simulink model "HFI_Test"  (R2023a)
settings: Solver=FixedStepAuto  StartTime=0.0  StopTime=1  FixedStep=Ts_simulink  RelTol=1e-3
model workspace (MATLAB code in the model file):
  | cmdLim = Simulink.Parameter;
  | cmdLim.Value = 15;
  | cmdLim.Description = 'Limit for controlling the maximum surface command angle.';
  | cmdLim.Min = 0;
  | cmdLim.Max = 90;
  | cmdLim.DocUnits = 'deg';
  | 
  | dispGain = Simulink.Parameter;
  | dispGain.Value = 0.75;
  | dispGain.Description = 'Gain applied to the displacement error.';
  | dispGain.Min = 0;
  | dispGain.Max = [];
  | dispGain.DocUnits = 'deg/sec/deg';
  | 
  | dispLim = Simulink.Parameter;
  | dispLim.Value = 30;
  | dispLim.Description = 'Limit for controlling the maximum commanded angle.';
  | dispLim.Min = 0;
  | dispLim.Max = 180;
  | dispLim.DocUnits = 'deg';
  | 
  | intGain = Simulink.Parameter;
  | intGain.Value = 0.5;
  | intGain.Description = 'Gain applied to the integral error.';
  | intGain.Min = 0;
  | intGain.Max = [];
  | intGain.DocUnits = 'deg/sec/deg/sec';
  | 
  | intLim = Simulink.Parameter;
  | intLim.Value = 5;
  | intLim.Description = 'Limit for controlling the maximum commanded angle.';
  | intLim.Min = 0;
  | intLim.Max = 90;
  | intLim.DocUnits = 'deg';
  | 
  | rateGain = Simulink.Parameter;
  | rateGain.Value = 2;
  | rateGain.Description = 'Gain applied to the rate error.';
  | rateGain.Min = 0;
  | rateGain.Max = [];
  | rateGain.DocUnits = 'deg/deg/sec';
  | 
  | rateLim = Simulink.Parameter;
  | rateLim.Value = 6;
  | rateLim.Description = 'Limit for controlling the maximum commanded angle.';
  | rateLim.Min = 0;
  | rateLim.Max = 180;
  | rateLim.DocUnits = 'deg/sec';
  | 
  | hdgGain = Simulink.Parameter;
  | hdgGain.Value = 0.015;
undefined symbols (not defined in the file): inverter, pmsm, Ts_motor, Ts_simulink
libraries: mcbcontrolslib x3, autolibpmsminterior x1, mcbplantlib x1
settings Model: RequirementInfo={} %GIDa_fe9045fd_0412_4b6e_8206_617cc20e6fde  Creator=洲  LastModifiedBy=洲
settings SolverCC: AlgebraicLoopSolver=TrustRegion  AutoInsertRateTranBlk=on
settings DataIOCC: SaveOutput=off  DSMLogging=off  SaveTime=off
settings OptimizationCC: DefaultParameterBehavior=Inlined  UseDivisionForNetSlopeComputation=on  GainParamInheritBuiltInType=on  UseFloatMulNetSlope=on  UseSpecifiedMinMax=on  InlineInvariantSignals=on  EnhancedBackFolding=on  PassReuseOutputArgsAs=Individual arguments  ZeroExternalMemoryAtStartup=off  ZeroInternalMemoryAtStartup=off  NoFixptDivByZeroProtection=on  EfficientFloat2IntCast=on  LifeSpan=1  OptimizeBlockOrder=speed  DifferentSizesBufferReuse=on  OptimizationCustomize=off  EfficientTunableParamExpr=on
settings DebuggingCC: AllowSymbolicDim=off  SFUnexpectedBacktrackingDiag=warning  SFNoUnconditionalDefaultTransitionDiag=warning  SFExecutionAtInitializationDiag=none  ArithmeticOperatorsInVariantConditions=warning
settings HardwareCC: ProdLongLongMode=on
settings SFSimCC: MATLABDynamicMemAlloc=off
settings RTWCC: Description=Embedded Coder  SystemTargetFile=ert.tlc  TemplateMakefile=ert_default_tmf  BuildConfiguration=Faster Runs  DataTypeReplacement=CDataTypesFixedWidth
settings CodeAppCC: ForceParamTrailComments=on  IgnoreCustomStorageClasses=off  OperatorAnnotations=on  SimulinkDataObjDesc=on  SFDataObjDesc=on  CustomSymbolStrGlobalVar=rt$N$M  CustomSymbolStrType=$N$M  CustomSymbolStrFcn=$N$M$F  CustomSymbolStrMacro=$N$M  InsertBlockDesc=on  EnableCustomComments=on  ReqsInCode=on
settings ERTTargetCC: TargetLangStandard=C99 (ISO)  UtilityFuncGeneration=Shared location  MultiwordLength=2048  GenerateSampleERTMain=on  IncludeMdlTerminateFcn=off  CombineSignalStateStructs=on  SuppressErrorStatus=on  SupportAbsoluteTime=off  SupportNonFinite=off  SupportComplex=off  InlinedParameterPlacement=NonHierarchical  ERTCustomFileTemplate=example_file_process.tlc  ERTFilePackagingFormat=CompactWithDataFile
settings ConfigComp: CovScope=ReferencedModels  CovSaveName=covdata_rollAP  CovMetricSettings=dcmtrwe  CovHTMLOptions=-sRT=1 -aTS=1 -bRG=1 -bTC=1 -hTR=1 -nFC=0 -scm=1 -bcm=1 -xEv=0  CovSaveCumulativeToWorkspaceVar=on  CovSaveSingleToWorkspaceVar=on  CovCumulativeVarName=covCumulativeData_rollAP  CovReportOnPause=off  CovExternalEMLEnable=off  CovSFcnEnable=off

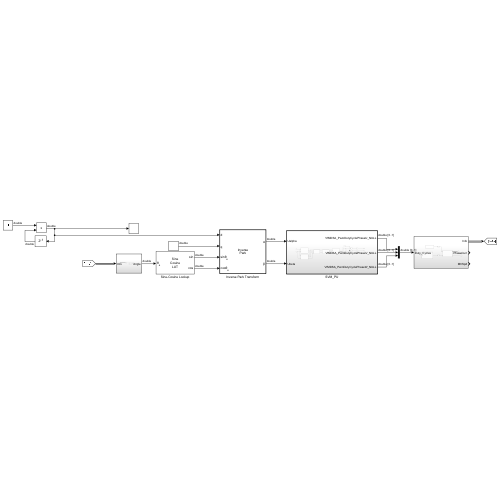
[thumbnail: Simulink's stored preview of the top-level diagram]
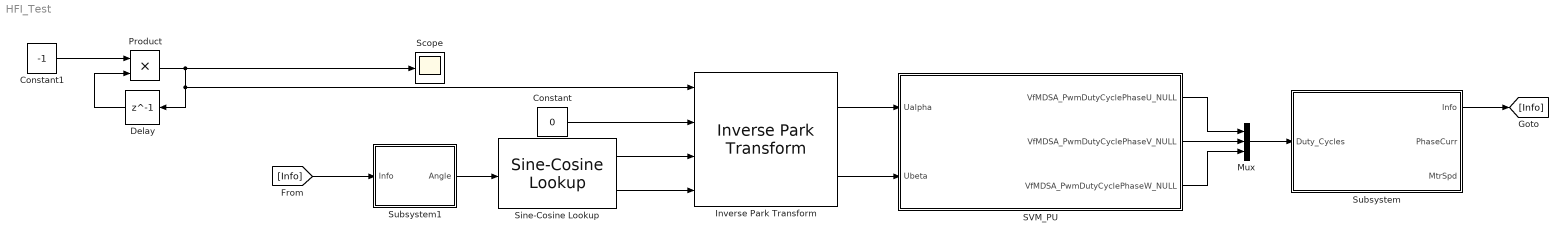
== system HFI_Test ==
  Constant : Constant  Value=0
  Constant1 : Constant  Value=-1  SampleTime=1e-4
  Delay : Delay  DelayLength=1  InitialCondition=3
  Inverse Park Transform : mcbcontrolslib/Inverse Park Transform  AxisAlignment=D-axis
      settings: LibrarySourceBlock=mcblib/Controls/Math Transforms/Inverse Park Transform
  Mux : Mux  Inputs=3
  Product : Product
  SVM_PU : Subsystem  TreatAsAtomicUnit=on  RTWFcnName=SVPWM_Calc
      settings: RTWSystemCode=Nonreusable function  RTWFcnNameOpts=User specified
  Scope : Scope
  Sine-Cosine Lookup : mcbcontrolslib/Sine-Cosine Lookup  AngleInput=Radians  N_points=4095
      settings: LibrarySourceBlock=mcblib/Controls/Math Transforms/Sine-Cosine Lookup
  Subsystem : Subsystem
  Subsystem1 : Subsystem
  wires:
  Mux/1 -> Subsystem/1(Duty_Cycles)
  SVM_PU/2(VfMDSA_PwmDutyCyclePhaseV_NULL) -> Mux/2
  SVM_PU/1(VfMDSA_PwmDutyCyclePhaseU_NULL) -> Mux/1
  SVM_PU/3(VfMDSA_PwmDutyCyclePhaseW_NULL) -> Mux/3
  Inverse Park Transform/1 -> SVM_PU/1(Ualpha)
  Inverse Park Transform/2 -> SVM_PU/2(Ubeta)
  Subsystem/1(Info) -> [Info]
  Sine-Cosine Lookup/2 -> Inverse Park Transform/4
  Sine-Cosine Lookup/1 -> Inverse Park Transform/3
  [Info] -> Subsystem1/1(Info)
  Subsystem1/1(Angle) -> Sine-Cosine Lookup/1
  Constant/1 -> Inverse Park Transform/2
  Product/1 -> Inverse Park Transform/1, Delay/1, Scope/1
  Delay/1 -> Product/2
  Constant1/1 -> Product/1

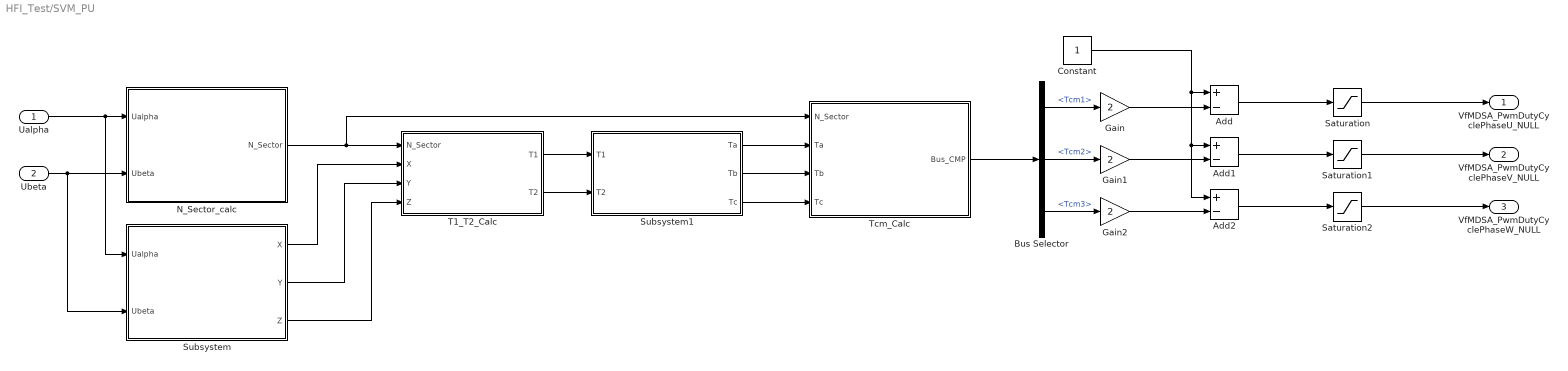
== system HFI_Test/SVM_PU ==
  Ualpha : Inport
  Ubeta : Inport  Port=2
  Add : Sum  Inputs=+-
  Add1 : Sum  Inputs=+-
  Add2 : Sum  Inputs=+-
  Bus Selector : BusSelector  OutputSignals=Tcm1,Tcm2,Tcm3
  Constant : Constant  OutDataTypeStr=single
  Gain : Gain  Gain=2
  Gain1 : Gain  Gain=2
  Gain2 : Gain  Gain=2
  N_Sector_calc : Subsystem
  Saturation : Saturate  UpperLimit=1  LowerLimit=0
  Saturation1 : Saturate  UpperLimit=1  LowerLimit=0
  Saturation2 : Saturate  UpperLimit=1  LowerLimit=0
  Subsystem : Subsystem
  Subsystem1 : Subsystem
  T1_T2_Calc : Subsystem
  Tcm_Calc : Subsystem
  VfMDSA_PwmDutyCyclePhaseU_NULL : Outport  OutMin=0  OutMax=1
  VfMDSA_PwmDutyCyclePhaseV_NULL : Outport  Port=2  OutMin=0  OutMax=1
  VfMDSA_PwmDutyCyclePhaseW_NULL : Outport  Port=3  OutMin=0  OutMax=1
  wires:
  Ualpha/1 -> Subsystem/1(Ualpha), N_Sector_calc/1(Ualpha)
  Ubeta/1 -> Subsystem/2(Ubeta), N_Sector_calc/2(Ubeta)
  N_Sector_calc/1(N_Sector) -> Tcm_Calc/1(N_Sector), T1_T2_Calc/1(N_Sector)
  Subsystem/1(X) -> T1_T2_Calc/2(X)
  Subsystem/2(Y) -> T1_T2_Calc/3(Y)
  Subsystem/3(Z) -> T1_T2_Calc/4(Z)
  Subsystem1/1(Ta) -> Tcm_Calc/2(Ta)
  Subsystem1/2(Tb) -> Tcm_Calc/3(Tb)
  Subsystem1/3(Tc) -> Tcm_Calc/4(Tc)
  Tcm_Calc/1(Bus_CMP) -> Bus Selector/1
  T1_T2_Calc/1(T1) -> Subsystem1/1(T1)
  T1_T2_Calc/2(T2) -> Subsystem1/2(T2)
  Bus Selector/1 -> Gain/1  "<Tcm1>"
  Bus Selector/2 -> Gain1/1  "<Tcm2>"
  Bus Selector/3 -> Gain2/1  "<Tcm3>"
  Constant/1 -> Add2/1, Add1/1, Add/1
  Gain/1 -> Add/2
  Gain1/1 -> Add1/2
  Gain2/1 -> Add2/2
  Add/1 -> Saturation/1
  Add1/1 -> Saturation1/1
  Add2/1 -> Saturation2/1
  Saturation/1 -> VfMDSA_PwmDutyCyclePhaseU_NULL/1
  Saturation1/1 -> VfMDSA_PwmDutyCyclePhaseV_NULL/1
  Saturation2/1 -> VfMDSA_PwmDutyCyclePhaseW_NULL/1

== system HFI_Test/Subsystem ==
  Duty_Cycles : Inport
  Interior PMSM : autolibpmsminterior/Interior PMSM  port_config=Torque  sim_type=Discrete  Ts=Ts_motor  P=4  Rs=0.02  Ldq=[1.7e-3 3.2e-3]  KConstText=Permanent flux linkage constant (lambda_pm):  lambda_pm=0.2205  Ke=159.9771  mechanical=[0.002700,4.924e-4,0]  idq0=[0 0]  theta_init=0  omega_init=0  KConst=0.2205  lambda_pm_calc=0.2205  Kt=0.07  RefBlkName='autolibpmsminterior/Interior PMSM'  aMode=5
      settings: LibrarySourceBlock=mcblib/Electrical Systems/Motors/Interior PMSM
  Inverter : Subsystem
  Load_Profile (Torque) : Subsystem
  Rate Transition : RateTransition  Deterministic=off  OutPortSampleTime=Ts_motor
  Rate Transition1 : RateTransition  Deterministic=off  OutPortSampleTime=Ts_motor
  Info : Outport
  PhaseCurr : Outport  Port=2
  MtrSpd : Outport  Port=3
  wires:
  Inverter/1(Vabc) -> Rate Transition/1  "Vabc"
  Rate Transition1/1 -> Interior PMSM/1
  Interior PMSM/3 -> MtrSpd/1
  Duty_Cycles/1 -> Inverter/1(Duty_abc)
  Rate Transition/1 -> Interior PMSM/2
  Interior PMSM/2 -> PhaseCurr/1  "Iabc"
  Load_Profile (Torque)/1(Load_Trq) -> Rate Transition1/1
  Interior PMSM/1 -> Info/1

== system HFI_Test/Subsystem1 ==
  Info : Inport
  Bus Selector : BusSelector  OutputSignals=MtrPos
  Constant : Constant  Value=2*pi
  Gain : Gain  Gain=4
  Mod : Math  Operator=mod
  Angle : Outport
  wires:
  Gain/1 -> Mod/1
  Mod/1 -> Angle/1
  Bus Selector/1 -> Gain/1  "<MtrPos>"
  Constant/1 -> Mod/2
  Info/1 -> Bus Selector/1

== system HFI_Test/SVM_PU/N_Sector_calc ==
  Ualpha : Inport
  Ubeta : Inport  Port=2
  N_calc : Subsystem
  Uref_Calc : Subsystem
  N_Sector : Outport
  wires:
  Uref_Calc/2(Uref2) -> N_calc/2(Uref2)
  Ualpha/1 -> Uref_Calc/1(Ualpha)
  Ubeta/1 -> Uref_Calc/2(Ubeta)
  Uref_Calc/3(Uref3) -> N_calc/3(Uref3)
  N_calc/1(N_Sector) -> N_Sector/1
  Uref_Calc/1(Uref1) -> N_calc/1(Uref1)

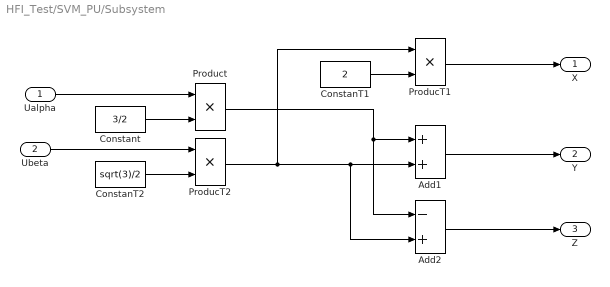
== system HFI_Test/SVM_PU/Subsystem ==
  Ualpha : Inport
  Ubeta : Inport  Port=2
  Add1 : Sum
  Add2 : Sum  Inputs=-+
  ConstanT1 : Constant  Value=2  OutDataTypeStr=single
  ConstanT2 : Constant  Value=sqrt(3)/2  OutDataTypeStr=single
  Constant : Constant  Value=3/2  OutDataTypeStr=single
  ProducT1 : Product
  ProducT2 : Product
  Product : Product
  X : Outport
  Y : Outport  Port=2
  Z : Outport  Port=3
  wires:
  Ualpha/1 -> Product/1
  Constant/1 -> Product/2
  ProducT1/1 -> X/1
  ConstanT1/1 -> ProducT1/2
  Ubeta/1 -> ProducT2/1
  Add1/1 -> Y/1
  Product/1 -> Add2/1, Add1/1
  ProducT2/1 -> ProducT1/1, Add2/2, Add1/2
  ConstanT2/1 -> ProducT2/2
  Add2/1 -> Z/1

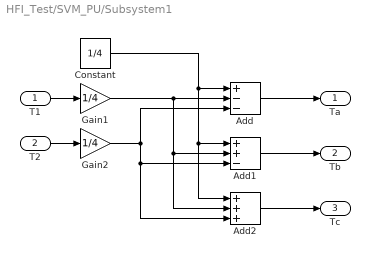
== system HFI_Test/SVM_PU/Subsystem1 ==
  T1 : Inport
  T2 : Inport  Port=2
  Add : Sum  Inputs=+--
  Add1 : Sum  Inputs=++-
  Add2 : Sum  Inputs=+++
  Constant : Constant  Value=1/4  OutDataTypeStr=single
  Gain1 : Gain  Gain=1/4
  Gain2 : Gain  Gain=1/4
  Ta : Outport
  Tb : Outport  Port=2
  Tc : Outport  Port=3
  wires:
  T1/1 -> Gain1/1
  T2/1 -> Gain2/1
  Constant/1 -> Add2/1, Add1/1, Add/1
  Add/1 -> Ta/1
  Gain1/1 -> Add2/2, Add1/2, Add/2
  Gain2/1 -> Add1/3, Add2/3, Add/3
  Add1/1 -> Tb/1
  Add2/1 -> Tc/1

== system HFI_Test/SVM_PU/T1_T2_Calc ==
  N_Sector : Inport
  X : Inport  Port=2
  Y : Inport  Port=3
  Z : Inport  Port=4
  Subsystem1 : Subsystem
  Subsystem2 : Subsystem
  T4_T6 : Subsystem  Commented=on
  T1 : Outport
  T2 : Outport  Port=2
  wires:
  X/1 -> Subsystem1/2(X)
  Z/1 -> Subsystem1/4(Z)
  N_Sector/1 -> Subsystem1/1(N_Sector)
  Y/1 -> Subsystem1/3(Y)
  Subsystem1/1(Bus_T4T6) -> Subsystem2/1(Bus_T4T6)
  Subsystem2/1(T1) -> T1/1
  Subsystem2/2(T2) -> T2/1

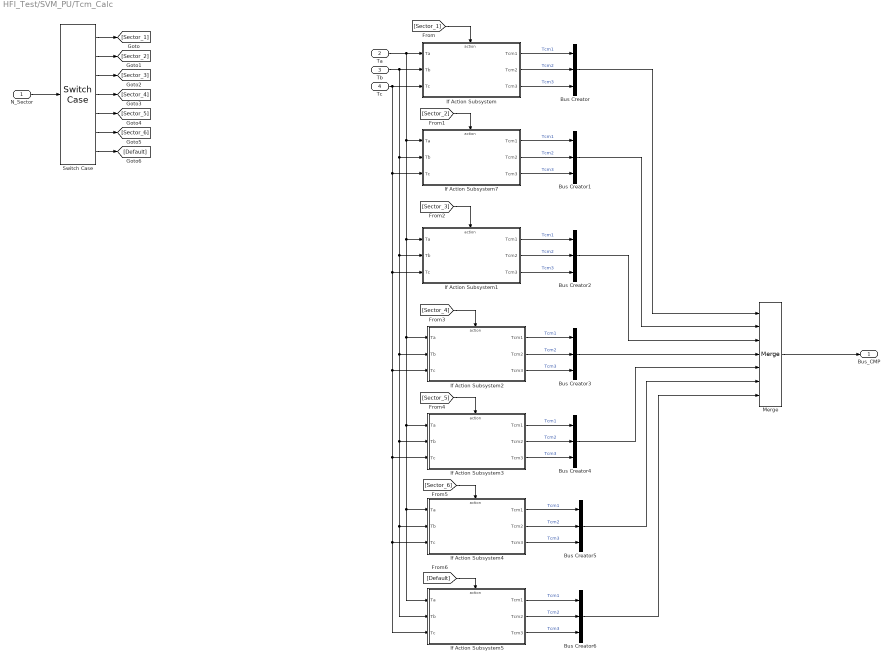
== system HFI_Test/SVM_PU/Tcm_Calc ==
  N_Sector : Inport
  Ta : Inport  Port=2
  Tb : Inport  Port=3
  Tc : Inport  Port=4
  Bus Creator{,1..6} (7 alike) : BusCreator  Inputs=3
  If Action Subsystem : Subsystem  TreatAsAtomicUnit=on
  If Action Subsystem1 : Subsystem  TreatAsAtomicUnit=on
  If Action Subsystem2 : Subsystem  TreatAsAtomicUnit=on
  If Action Subsystem3 : Subsystem  TreatAsAtomicUnit=on
  If Action Subsystem4 : Subsystem  TreatAsAtomicUnit=on
  If Action Subsystem5 : Subsystem  TreatAsAtomicUnit=on
  If Action Subsystem7 : Subsystem  TreatAsAtomicUnit=on
  Merge : Merge  Inputs=7
  Switch Case : SwitchCase  CaseConditions={1,2,3,4,5,6}
  Bus_CMP : Outport
  wires:
  Switch Case/1 -> [Sector_1]
  Switch Case/2 -> [Sector_2]
  Switch Case/4 -> [Sector_4]
  Switch Case/6 -> [Sector_6]
  Switch Case/3 -> [Sector_3]
  N_Sector/1 -> Switch Case/1
  Switch Case/7 -> [Default]
  Switch Case/5 -> [Sector_5]
  [Sector_1] -> If Action Subsystem/Action
  [Sector_2] -> If Action Subsystem7/Action
  [Sector_4] -> If Action Subsystem2/Action
  [Sector_3] -> If Action Subsystem1/Action
  [Sector_6] -> If Action Subsystem4/Action
  [Sector_5] -> If Action Subsystem3/Action
  [Default] -> If Action Subsystem5/Action
  Tb/1 -> If Action Subsystem5/2(Tb), If Action Subsystem4/2(Tb), If Action Subsystem3/2(Tb), If Action Subsystem2/2(Tb), If Action Subsystem1/2(Tb), If Action Subsystem7/2(Tb), If Action Subsystem/2(Tb)
  Tc/1 -> If Action Subsystem/3(Tc), If Action Subsystem5/3(Tc), If Action Subsystem4/3(Tc), If Action Subsystem3/3(Tc), If Action Subsystem2/3(Tc), If Action Subsystem1/3(Tc), If Action Subsystem7/3(Tc)
  Ta/1 -> If Action Subsystem5/1(Ta), If Action Subsystem4/1(Ta), If Action Subsystem3/1(Ta), If Action Subsystem2/1(Ta), If Action Subsystem1/1(Ta), If Action Subsystem7/1(Ta), If Action Subsystem/1(Ta)
  Merge/1 -> Bus_CMP/1
  If Action Subsystem/1(Tcm1) -> Bus Creator/1  "Tcm1"
  If Action Subsystem/2(Tcm2) -> Bus Creator/2  "Tcm2"
  If Action Subsystem/3(Tcm3) -> Bus Creator/3  "Tcm3"
  If Action Subsystem7/1(Tcm1) -> Bus Creator1/1  "Tcm1"
  If Action Subsystem7/3(Tcm3) -> Bus Creator1/3  "Tcm3"
  If Action Subsystem7/2(Tcm2) -> Bus Creator1/2  "Tcm2"
  If Action Subsystem1/1(Tcm1) -> Bus Creator2/1  "Tcm1"
  If Action Subsystem1/3(Tcm3) -> Bus Creator2/3  "Tcm3"
  If Action Subsystem1/2(Tcm2) -> Bus Creator2/2  "Tcm2"
  If Action Subsystem2/1(Tcm1) -> Bus Creator3/1  "Tcm1"
  If Action Subsystem2/3(Tcm3) -> Bus Creator3/3  "Tcm3"
  If Action Subsystem2/2(Tcm2) -> Bus Creator3/2  "Tcm2"
  If Action Subsystem3/1(Tcm1) -> Bus Creator4/1  "Tcm1"
  If Action Subsystem3/3(Tcm3) -> Bus Creator4/3  "Tcm3"
  If Action Subsystem3/2(Tcm2) -> Bus Creator4/2  "Tcm2"
  If Action Subsystem4/1(Tcm1) -> Bus Creator5/1  "Tcm1"
  If Action Subsystem4/3(Tcm3) -> Bus Creator5/3  "Tcm3"
  If Action Subsystem4/2(Tcm2) -> Bus Creator5/2  "Tcm2"
  If Action Subsystem5/1(Tcm1) -> Bus Creator6/1  "Tcm1"
  If Action Subsystem5/3(Tcm3) -> Bus Creator6/3  "Tcm3"
  If Action Subsystem5/2(Tcm2) -> Bus Creator6/2  "Tcm2"
  Bus Creator/1 -> Merge/1
  Bus Creator1/1 -> Merge/2
  Bus Creator2/1 -> Merge/3
  Bus Creator3/1 -> Merge/4
  Bus Creator4/1 -> Merge/5
  Bus Creator5/1 -> Merge/6
  Bus Creator6/1 -> Merge/7

== system HFI_Test/Subsystem/Inverter ==
  Duty_abc : Inport
  Average-Value Inverter : mcbplantlib/Average-Value Inverter
  Constant2 : Constant  Value=inverter.V_dc  OutDataTypeStr=single  SampleTime=-1
  Data Type Conversion1 : DataTypeConversion  OutDataTypeStr=single  RndMeth=Simplest  SaturateOnIntegerOverflow=off
  Rate Transition3 : RateTransition  Deterministic=off  OutPortSampleTime=Ts_inverter
  Vabc : Outport  VectorParamsAs1DForOutWhenUnconnected=off
  wires:
  Constant2/1 -> Average-Value Inverter/2
  Data Type Conversion1/1 -> Rate Transition3/1
  Duty_abc/1 -> Data Type Conversion1/1
  Average-Value Inverter/1 -> Vabc/1
  Rate Transition3/1 -> Average-Value Inverter/1

== system HFI_Test/Subsystem/Load_Profile (Torque) ==
  Constant : Constant  Value=0
  Data Type Conversion : DataTypeConversion  OutDataTypeStr=single  SaturateOnIntegerOverflow=off  RndMeth=Floor
  IIR Filter : mcbcontrolslib/IIR Filter  VariantControl=Low Pass Filter  VariantSelect=Low-pass  Filter_constant=0.0001  advancedSettings=off  Ts=50e-6  cutOff_freq=0.31834
  T_load : Step  Commented=on  Time=4  Before=0.05*pmsm.T_rated  After=0.5*pmsm.T_rated  SampleTime=Ts_simulink
  Load_Trq : Outport  VectorParamsAs1DForOutWhenUnconnected=off
  wires:
  Data Type Conversion/1 -> IIR Filter/1
  IIR Filter/1 -> Load_Trq/1
  Constant/1 -> Data Type Conversion/1

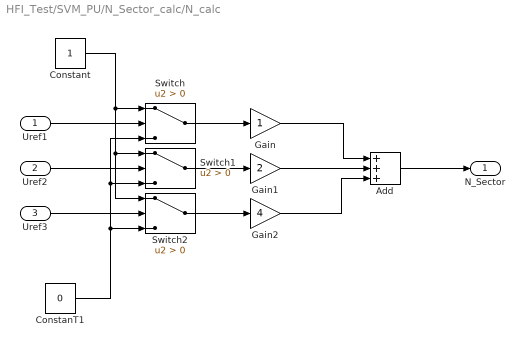
== system HFI_Test/SVM_PU/N_Sector_calc/N_calc ==
  Uref1 : Inport
  Uref2 : Inport  Port=2
  Uref3 : Inport  Port=3
  Add : Sum  Inputs=+++
  ConstanT1 : Constant  Value=0  OutDataTypeStr=single
  Constant : Constant  OutDataTypeStr=single
  Gain : Gain
  Gain1 : Gain  Gain=2
  Gain2 : Gain  Gain=4
  Switch : Switch  Criteria=u2 > Threshold  SaturateOnIntegerOverflow=off  InputSameDT=off
  Switch1 : Switch  Criteria=u2 > Threshold  SaturateOnIntegerOverflow=off  InputSameDT=off
  Switch2 : Switch  Criteria=u2 > Threshold  SaturateOnIntegerOverflow=off  InputSameDT=off
  N_Sector : Outport
  wires:
  Uref1/1 -> Switch/2
  Uref2/1 -> Switch1/2
  Uref3/1 -> Switch2/2
  ConstanT1/1 -> Switch2/3, Switch/3, Switch1/3
  Constant/1 -> Switch2/1, Switch1/1, Switch/1
  Switch1/1 -> Gain1/1
  Switch/1 -> Gain/1
  Switch2/1 -> Gain2/1
  Add/1 -> N_Sector/1
  Gain/1 -> Add/1
  Gain1/1 -> Add/2
  Gain2/1 -> Add/3

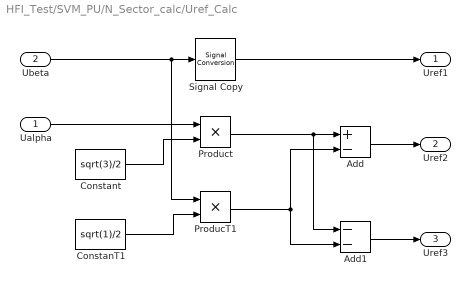
== system HFI_Test/SVM_PU/N_Sector_calc/Uref_Calc ==
  Ualpha : Inport
  Ubeta : Inport  Port=2
  Add : Sum  Inputs=+-
  Add1 : Sum  Inputs=--
  ConstanT1 : Constant  Value=sqrt(1)/2  OutDataTypeStr=single
  Constant : Constant  Value=sqrt(3)/2  OutDataTypeStr=single
  ProducT1 : Product
  Product : Product
  Signal Copy : SignalConversion  OverrideOpt=off
  Uref1 : Outport
  Uref2 : Outport  Port=2
  Uref3 : Outport  Port=3
  wires:
  Ubeta/1 -> ProducT1/1, Signal Copy/1
  Signal Copy/1 -> Uref1/1
  Ualpha/1 -> Product/1
  Constant/1 -> Product/2
  ConstanT1/1 -> ProducT1/2
  Product/1 -> Add1/1, Add/1
  ProducT1/1 -> Add1/2, Add/2
  Add/1 -> Uref2/1
  Add1/1 -> Uref3/1

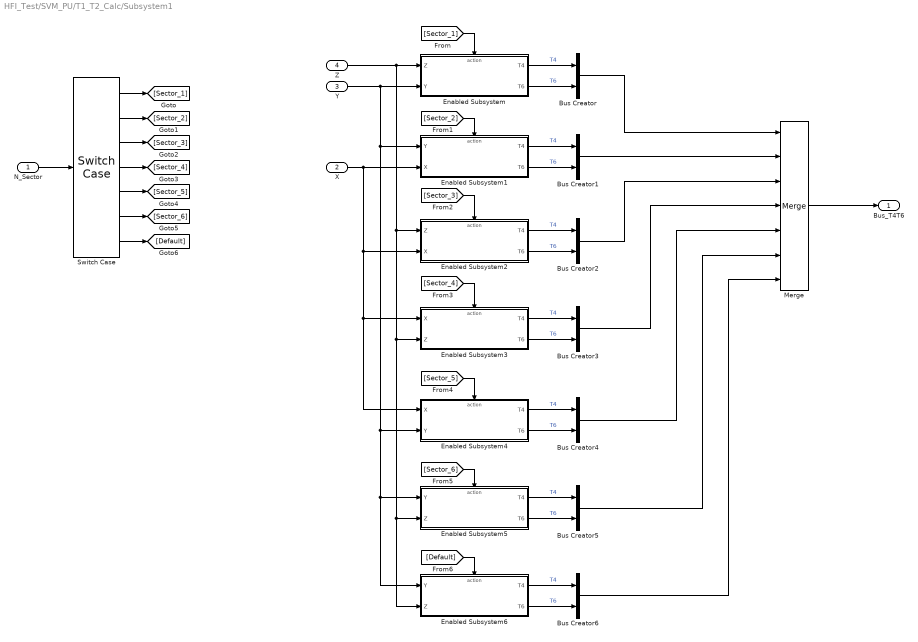
== system HFI_Test/SVM_PU/T1_T2_Calc/Subsystem1 ==
  N_Sector : Inport
  X : Inport  Port=2
  Y : Inport  Port=3
  Z : Inport  Port=4
  Bus Creator{,1..6} (7 alike) : BusCreator  Inputs=2
  Enabled Subsystem : Subsystem  TreatAsAtomicUnit=on
  Enabled Subsystem1 : Subsystem  TreatAsAtomicUnit=on
  Enabled Subsystem2 : Subsystem  TreatAsAtomicUnit=on
  Enabled Subsystem3 : Subsystem  TreatAsAtomicUnit=on
  Enabled Subsystem4 : Subsystem  TreatAsAtomicUnit=on
  Enabled Subsystem5 : Subsystem  TreatAsAtomicUnit=on
  Enabled Subsystem6 : Subsystem  TreatAsAtomicUnit=on
  Merge : Merge  Inputs=7
  Switch Case : SwitchCase  CaseConditions={1,2,3,4,5,6}
  Bus_T4T6 : Outport
  wires:
  N_Sector/1 -> Switch Case/1
  Switch Case/1 -> [Sector_1]
  Switch Case/2 -> [Sector_2]
  Switch Case/3 -> [Sector_3]
  Switch Case/4 -> [Sector_4]
  Switch Case/5 -> [Sector_5]
  Switch Case/6 -> [Sector_6]
  Switch Case/7 -> [Default]
  [Sector_1] -> Enabled Subsystem/Action
  Y/1 -> Enabled Subsystem6/1(Y), Enabled Subsystem5/1(Y), Enabled Subsystem4/2(Y), Enabled Subsystem1/1(Y), Enabled Subsystem/2(Y)
  Z/1 -> Enabled Subsystem3/2(Z), Enabled Subsystem6/2(Z), Enabled Subsystem5/2(Z), Enabled Subsystem2/1(Z), Enabled Subsystem/1(Z)
  [Sector_2] -> Enabled Subsystem1/Action
  X/1 -> Enabled Subsystem4/1(X), Enabled Subsystem3/1(X), Enabled Subsystem2/2(X), Enabled Subsystem1/2(X)
  [Sector_3] -> Enabled Subsystem2/Action
  [Sector_4] -> Enabled Subsystem3/Action
  [Sector_5] -> Enabled Subsystem4/Action
  [Sector_6] -> Enabled Subsystem5/Action
  [Default] -> Enabled Subsystem6/Action
  Enabled Subsystem/1(T4) -> Bus Creator/1  "T4"
  Enabled Subsystem/2(T6) -> Bus Creator/2  "T6"
  Enabled Subsystem1/2(T6) -> Bus Creator1/2  "T6"
  Enabled Subsystem1/1(T4) -> Bus Creator1/1  "T4"
  Enabled Subsystem2/1(T4) -> Bus Creator2/1  "T4"
  Enabled Subsystem3/1(T4) -> Bus Creator3/1  "T4"
  Enabled Subsystem2/2(T6) -> Bus Creator2/2  "T6"
  Enabled Subsystem3/2(T6) -> Bus Creator3/2  "T6"
  Enabled Subsystem4/1(T4) -> Bus Creator4/1  "T4"
  Enabled Subsystem5/1(T4) -> Bus Creator5/1  "T4"
  Enabled Subsystem4/2(T6) -> Bus Creator4/2  "T6"
  Enabled Subsystem5/2(T6) -> Bus Creator5/2  "T6"
  Enabled Subsystem6/1(T4) -> Bus Creator6/1  "T4"
  Enabled Subsystem6/2(T6) -> Bus Creator6/2  "T6"
  Bus Creator/1 -> Merge/1
  Bus Creator1/1 -> Merge/2
  Bus Creator2/1 -> Merge/3
  Bus Creator3/1 -> Merge/4
  Bus Creator4/1 -> Merge/5
  Bus Creator5/1 -> Merge/6
  Bus Creator6/1 -> Merge/7
  Merge/1 -> Bus_T4T6/1

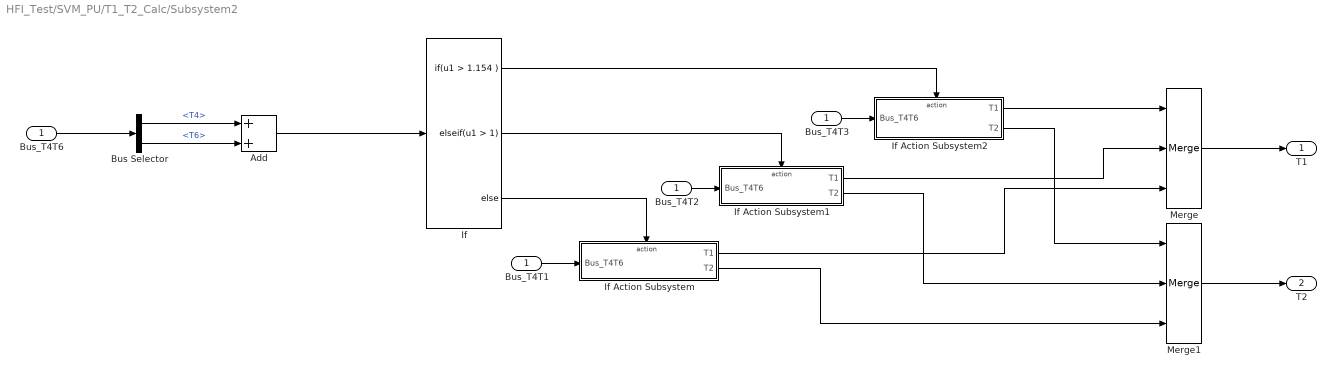
== system HFI_Test/SVM_PU/T1_T2_Calc/Subsystem2 ==
  Bus_T4T6 : Inport
  Add : Sum
  Bus Selector : BusSelector  OutputSignals=T4,T6
  Bus_T4T1 : InportShadow
  Bus_T4T2 : InportShadow
  Bus_T4T3 : InportShadow
  If : If  IfExpression=u1 > 1.154  ElseIfExpressions=u1 > 1
  If Action Subsystem : Subsystem  TreatAsAtomicUnit=on
  If Action Subsystem1 : Subsystem  TreatAsAtomicUnit=on
  If Action Subsystem2 : Subsystem  TreatAsAtomicUnit=on
  Merge : Merge  Inputs=3
  Merge1 : Merge  Inputs=3
  T1 : Outport
  T2 : Outport  Port=2
  wires:
  Bus_T4T6/1 -> Bus Selector/1
  Bus Selector/1 -> Add/1  "<T4>"
  Bus Selector/2 -> Add/2  "<T6>"
  Add/1 -> If/1
  If/3 -> If Action Subsystem/Action
  If/2 -> If Action Subsystem1/Action
  If/1 -> If Action Subsystem2/Action
  Bus_T4T1/1 -> If Action Subsystem/1(Bus_T4T6)
  Bus_T4T2/1 -> If Action Subsystem1/1(Bus_T4T6)
  Bus_T4T3/1 -> If Action Subsystem2/1(Bus_T4T6)
  Merge/1 -> T1/1
  If Action Subsystem2/1(T1) -> Merge/1
  If Action Subsystem1/1(T1) -> Merge/2
  If Action Subsystem/1(T1) -> Merge/3
  If Action Subsystem2/2(T2) -> Merge1/1
  If Action Subsystem1/2(T2) -> Merge1/2
  If Action Subsystem/2(T2) -> Merge1/3
  Merge1/1 -> T2/1

== system HFI_Test/SVM_PU/T1_T2_Calc/T4_T6 ==
  T4 : Inport
  T6 : Inport  Port=2
  Add : Sum
  Divide : Product  Inputs=*/
  Divide1 : Product  Inputs=*/
  Mux : Mux  Inputs=2
  Mux1 : Mux  Inputs=2
  Switch : Switch  Criteria=u2 > Threshold  Threshold=1  SaturateOnIntegerOverflow=off  InputSameDT=off
  T4_T6 : Outport
  wires:
  T4/1 -> Add/1, Mux1/1, Divide/1
  T6/1 -> Mux1/2, Add/2, Divide1/1
  Add/1 -> Divide1/2, Divide/2, Switch/2
  Divide/1 -> Mux/1  "T4"
  Divide1/1 -> Mux/2  "T6"
  Mux/1 -> Switch/1
  Mux1/1 -> Switch/3
  Switch/1 -> T4_T6/1

== system HFI_Test/SVM_PU/Tcm_Calc/If Action Subsystem ==
  Ta : Inport
  Tb : Inport  Port=2
  Tc : Inport  Port=3
  Action Port : ActionPort  ActionPortLabel=case [ 1 ]:
  Tcm1 : Outport
  Tcm2 : Outport  Port=2
  Tcm3 : Outport  Port=3
  wires:
  Tb/1 -> Tcm1/1
  Ta/1 -> Tcm2/1
  Tc/1 -> Tcm3/1

== system HFI_Test/SVM_PU/Tcm_Calc/If Action Subsystem1 ==
  Ta : Inport
  Tb : Inport  Port=2
  Tc : Inport  Port=3
  Action Port : ActionPort  ActionPortLabel=case [ 3 ]:
  Tcm1 : Outport
  Tcm2 : Outport  Port=2
  Tcm3 : Outport  Port=3
  wires:
  Ta/1 -> Tcm1/1
  Tb/1 -> Tcm2/1
  Tc/1 -> Tcm3/1

== system HFI_Test/SVM_PU/Tcm_Calc/If Action Subsystem2 ==
  Ta : Inport
  Tb : Inport  Port=2
  Tc : Inport  Port=3
  Action Port : ActionPort  ActionPortLabel=case [ 4 ]:
  Tcm1 : Outport
  Tcm2 : Outport  Port=2
  Tcm3 : Outport  Port=3
  wires:
  Tc/1 -> Tcm1/1
  Tb/1 -> Tcm2/1
  Ta/1 -> Tcm3/1

== system HFI_Test/SVM_PU/Tcm_Calc/If Action Subsystem3 ==
  Ta : Inport
  Tb : Inport  Port=2
  Tc : Inport  Port=3
  Action Port : ActionPort  ActionPortLabel=case [ 5 ]:
  Tcm1 : Outport
  Tcm2 : Outport  Port=2
  Tcm3 : Outport  Port=3
  wires:
  Tc/1 -> Tcm1/1
  Tb/1 -> Tcm3/1
  Ta/1 -> Tcm2/1

== system HFI_Test/SVM_PU/Tcm_Calc/If Action Subsystem4 ==
  Ta : Inport
  Tb : Inport  Port=2
  Tc : Inport  Port=3
  Action Port : ActionPort  ActionPortLabel=case [ 6 ]:
  Tcm1 : Outport
  Tcm2 : Outport  Port=2
  Tcm3 : Outport  Port=3
  wires:
  Tc/1 -> Tcm2/1
  Tb/1 -> Tcm1/1
  Ta/1 -> Tcm3/1

== system HFI_Test/SVM_PU/Tcm_Calc/If Action Subsystem5 ==
  Ta : Inport
  Tb : Inport  Port=2
  Tc : Inport  Port=3
  Action Port : ActionPort  ActionPortLabel=default:
  Tcm1 : Outport
  Tcm2 : Outport  Port=2
  Tcm3 : Outport  Port=3
  wires:
  Tc/1 -> Tcm2/1
  Tb/1 -> Tcm1/1
  Ta/1 -> Tcm3/1

== system HFI_Test/SVM_PU/Tcm_Calc/If Action Subsystem7 ==
  Ta : Inport
  Tb : Inport  Port=2
  Tc : Inport  Port=3
  Action Port : ActionPort  ActionPortLabel=case [ 2 ]:
  Tcm1 : Outport
  Tcm2 : Outport  Port=2
  Tcm3 : Outport  Port=3
  wires:
  Ta/1 -> Tcm1/1
  Tc/1 -> Tcm2/1
  Tb/1 -> Tcm3/1

== system HFI_Test/SVM_PU/T1_T2_Calc/Subsystem1/Enabled Subsystem ==
  Z : Inport
  Y : Inport  Port=2
  Action Port : ActionPort  ActionPortLabel=case [ 1 ]:
  T4 : Outport
  T6 : Outport  Port=2
  wires:
  Z/1 -> T4/1
  Y/1 -> T6/1

== system HFI_Test/SVM_PU/T1_T2_Calc/Subsystem1/Enabled Subsystem1 ==
  Y : Inport
  X : Inport  Port=2
  Action Port : ActionPort  ActionPortLabel=case [ 2 ]:
  Gain : Gain  Gain=-1
  T4 : Outport
  T6 : Outport  Port=2
  wires:
  Y/1 -> T4/1
  Gain/1 -> T6/1
  X/1 -> Gain/1

== system HFI_Test/SVM_PU/T1_T2_Calc/Subsystem1/Enabled Subsystem2 ==
  Z : Inport
  X : Inport  Port=2
  Action Port : ActionPort  ActionPortLabel=case [ 3 ]:
  Gain : Gain  Gain=-1
  T4 : Outport
  T6 : Outport  Port=2
  wires:
  Z/1 -> Gain/1
  X/1 -> T6/1
  Gain/1 -> T4/1

== system HFI_Test/SVM_PU/T1_T2_Calc/Subsystem1/Enabled Subsystem3 ==
  X : Inport
  Z : Inport  Port=2
  Action Port : ActionPort  ActionPortLabel=case [ 4 ]:
  Gain : Gain  Gain=-1
  T4 : Outport
  T6 : Outport  Port=2
  wires:
  X/1 -> Gain/1
  Z/1 -> T6/1
  Gain/1 -> T4/1

== system HFI_Test/SVM_PU/T1_T2_Calc/Subsystem1/Enabled Subsystem4 ==
  X : Inport
  Y : Inport  Port=2
  Action Port : ActionPort  ActionPortLabel=case [ 5 ]:
  Gain : Gain  Gain=-1
  T4 : Outport
  T6 : Outport  Port=2
  wires:
  Y/1 -> Gain/1
  X/1 -> T4/1
  Gain/1 -> T6/1

== system HFI_Test/SVM_PU/T1_T2_Calc/Subsystem1/Enabled Subsystem5 ==
  Y : Inport
  Z : Inport  Port=2
  Action Port : ActionPort  ActionPortLabel=case [ 6 ]:
  Gain : Gain  Gain=-1
  Gain1 : Gain  Gain=-1
  T4 : Outport
  T6 : Outport  Port=2
  wires:
  Y/1 -> Gain/1
  Z/1 -> Gain1/1
  Gain/1 -> T4/1
  Gain1/1 -> T6/1

== system HFI_Test/SVM_PU/T1_T2_Calc/Subsystem1/Enabled Subsystem6 ==
  Y : Inport
  Z : Inport  Port=2
  Action Port : ActionPort  ActionPortLabel=default:
  Gain : Gain  Gain=-1
  Gain1 : Gain  Gain=-1
  T4 : Outport
  T6 : Outport  Port=2
  wires:
  Y/1 -> Gain/1
  Z/1 -> Gain1/1
  Gain/1 -> T4/1
  Gain1/1 -> T6/1

== system HFI_Test/SVM_PU/T1_T2_Calc/Subsystem2/If Action Subsystem ==
  Bus_T4T6 : Inport
  Action Port : ActionPort  ActionPortLabel=else
  Bus Selector : BusSelector  OutputSignals=T4,T6
  Signal Copy1 : SignalConversion  OverrideOpt=off
  Signal Copy2 : SignalConversion  OverrideOpt=off
  T1 : Outport
  T2 : Outport  Port=2
  wires:
  Bus_T4T6/1 -> Bus Selector/1
  Bus Selector/1 -> Signal Copy1/1  "<T4>"
  Bus Selector/2 -> Signal Copy2/1  "<T6>"
  Signal Copy1/1 -> T1/1
  Signal Copy2/1 -> T2/1

== system HFI_Test/SVM_PU/T1_T2_Calc/Subsystem2/If Action Subsystem1 ==
  Bus_T4T6 : Inport
  Action Port : ActionPort  ActionPortLabel=elseif(u1 > 1)
  Add : Sum
  Bus Selector : BusSelector  OutputSignals=T4,T6
  Divide : Product  Inputs=*/
  Divide1 : Product  Inputs=/*
  T1 : Outport
  T2 : Outport  Port=2
  wires:
  Bus_T4T6/1 -> Bus Selector/1
  Bus Selector/1 -> Divide/1, Add/1  "<T4>"
  Bus Selector/2 -> Divide1/2, Add/2  "<T6>"
  Add/1 -> Divide1/1, Divide/2
  Divide/1 -> T1/1  "T1"
  Divide1/1 -> T2/1  "T2"

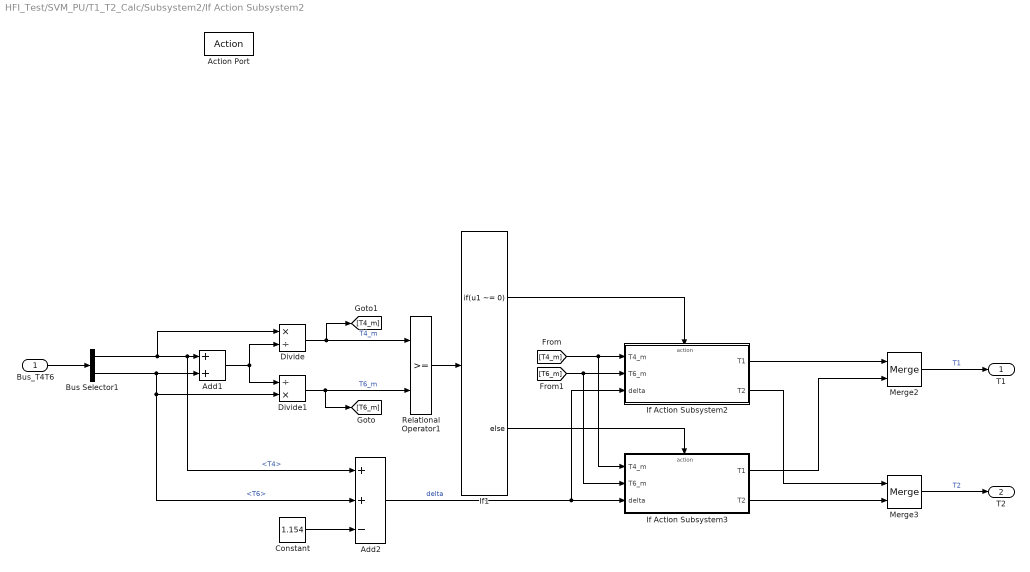
== system HFI_Test/SVM_PU/T1_T2_Calc/Subsystem2/If Action Subsystem2 ==
  Bus_T4T6 : Inport
  Action Port : ActionPort  ActionPortLabel=if(u1 > 1.154 )
  Add1 : Sum
  Add2 : Sum  Inputs=++-
  Bus Selector1 : BusSelector  OutputSignals=T4,T6
  Constant : Constant  Value=1.154  OutDataTypeStr=single
  Divide : Product  Inputs=*/
  Divide1 : Product  Inputs=/*
  If Action Subsystem2 : Subsystem  TreatAsAtomicUnit=on
  If Action Subsystem3 : Subsystem  TreatAsAtomicUnit=on
  If1 : If  IfExpression=u1 ~= 0
  Merge2 : Merge
  Merge3 : Merge
  Relational Operator1 : RelationalOperator  OutDataTypeStr=boolean  RndMeth=Simplest  InputSameDT=off
  T1 : Outport
  T2 : Outport  Port=2
  wires:
  Bus_T4T6/1 -> Bus Selector1/1
  Bus Selector1/2 -> Divide1/2, Add2/2, Add1/2  "<T6>"
  Divide/1 -> [T4_m], Relational Operator1/1  "T4_m"
  Bus Selector1/1 -> Divide/1, Add2/1, Add1/1  "<T4>"
  Divide1/1 -> [T6_m], Relational Operator1/2  "T6_m"
  Add1/1 -> Divide1/1, Divide/2
  Relational Operator1/1 -> If1/1
  Constant/1 -> Add2/3
  Add2/1 -> If Action Subsystem2/3(delta), If Action Subsystem3/3(delta)  "delta"
  If1/1 -> If Action Subsystem2/Action
  If1/2 -> If Action Subsystem3/Action
  If Action Subsystem2/1(T1) -> Merge2/1
  If Action Subsystem3/1(T1) -> Merge2/2
  If Action Subsystem3/2(T2) -> Merge3/2
  If Action Subsystem2/2(T2) -> Merge3/1
  Merge2/1 -> T1/1  "T1"
  Merge3/1 -> T2/1  "T2"
  [T4_m] -> If Action Subsystem3/1(T4_m), If Action Subsystem2/1(T4_m)
  [T6_m] -> If Action Subsystem3/2(T6_m), If Action Subsystem2/2(T6_m)

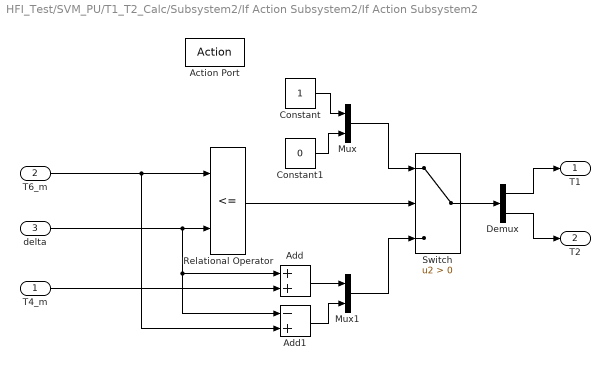
== system HFI_Test/SVM_PU/T1_T2_Calc/Subsystem2/If Action Subsystem2/If Action Subsystem2 ==
  T4_m : Inport
  T6_m : Inport  Port=2
  delta : Inport  Port=3
  Action Port : ActionPort  ActionPortLabel=if(u1 ~= 0)
  Add : Sum
  Add1 : Sum  Inputs=-+
  Constant : Constant  OutDataTypeStr=single
  Constant1 : Constant  Value=0  OutDataTypeStr=single
  Demux : Demux  Outputs=2
  Mux : Mux  Inputs=2
  Mux1 : Mux  Inputs=2
  Relational Operator : RelationalOperator  Operator=<=  OutDataTypeStr=boolean  RndMeth=Simplest  InputSameDT=off
  Switch : Switch  Criteria=u2 > Threshold  SaturateOnIntegerOverflow=off  InputSameDT=off
  T1 : Outport
  T2 : Outport  Port=2
  wires:
  T6_m/1 -> Add1/2, Relational Operator/1
  delta/1 -> Add/1, Add1/1, Relational Operator/2
  Relational Operator/1 -> Switch/2
  Constant/1 -> Mux/1
  Constant1/1 -> Mux/2
  Mux/1 -> Switch/1
  T4_m/1 -> Add/2
  Add/1 -> Mux1/1
  Add1/1 -> Mux1/2
  Mux1/1 -> Switch/3
  Switch/1 -> Demux/1
  Demux/1 -> T1/1
  Demux/2 -> T2/1

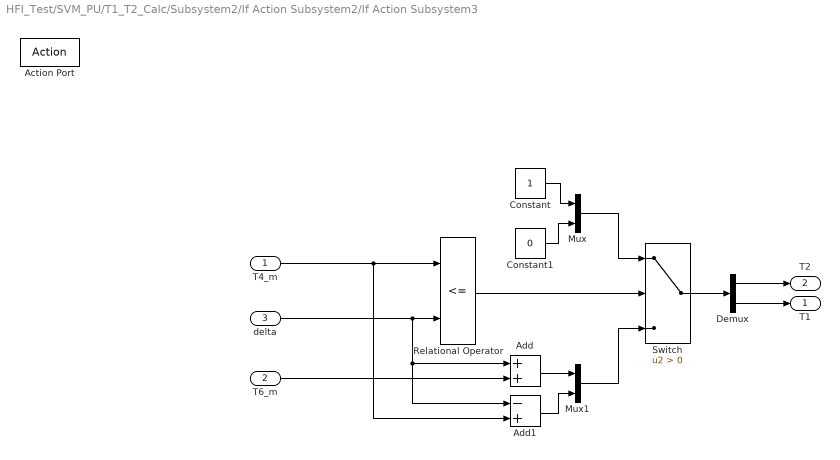
== system HFI_Test/SVM_PU/T1_T2_Calc/Subsystem2/If Action Subsystem2/If Action Subsystem3 ==
  T4_m : Inport
  T6_m : Inport  Port=2
  delta : Inport  Port=3
  Action Port : ActionPort  ActionPortLabel=else
  Add : Sum
  Add1 : Sum  Inputs=-+
  Constant : Constant  OutDataTypeStr=single
  Constant1 : Constant  Value=0  OutDataTypeStr=single
  Demux : Demux  Outputs=2
  Mux : Mux  Inputs=2
  Mux1 : Mux  Inputs=2
  Relational Operator : RelationalOperator  Operator=<=  OutDataTypeStr=boolean  RndMeth=Simplest  InputSameDT=off
  Switch : Switch  Criteria=u2 > Threshold  SaturateOnIntegerOverflow=off  InputSameDT=off
  T1 : Outport
  T2 : Outport  Port=2
  wires:
  Mux1/1 -> Switch/3
  delta/1 -> Add/1, Add1/1, Relational Operator/2
  Add1/1 -> Mux1/2
  Mux/1 -> Switch/1
  Relational Operator/1 -> Switch/2
  Switch/1 -> Demux/1
  Constant1/1 -> Mux/2
  Add/1 -> Mux1/1
  Constant/1 -> Mux/1
  T4_m/1 -> Add1/2, Relational Operator/1
  T6_m/1 -> Add/2
  Demux/2 -> T1/1
  Demux/1 -> T2/1
